simulink model "test_1"  (Simulink 8.9)
settings: Solver=FixedStepAuto  StartTime=0.0  StopTime=inf  RelTol=1e-3  EnableMultiTasking=on
libraries: Solver_SF x1, sldrtlib x1, simulink x1
settings Model: Creator=anan  ModifiedByFormat=an  LastModifiedBy=an
settings DataIOCC: ExternalInput=[t, input_1]  SignalLoggingSaveFormat=Dataset
settings OptimizationCC: ExpressionDepthLimit=2147483647
settings DebuggingCC: SolverPrmCheckMsg=warning

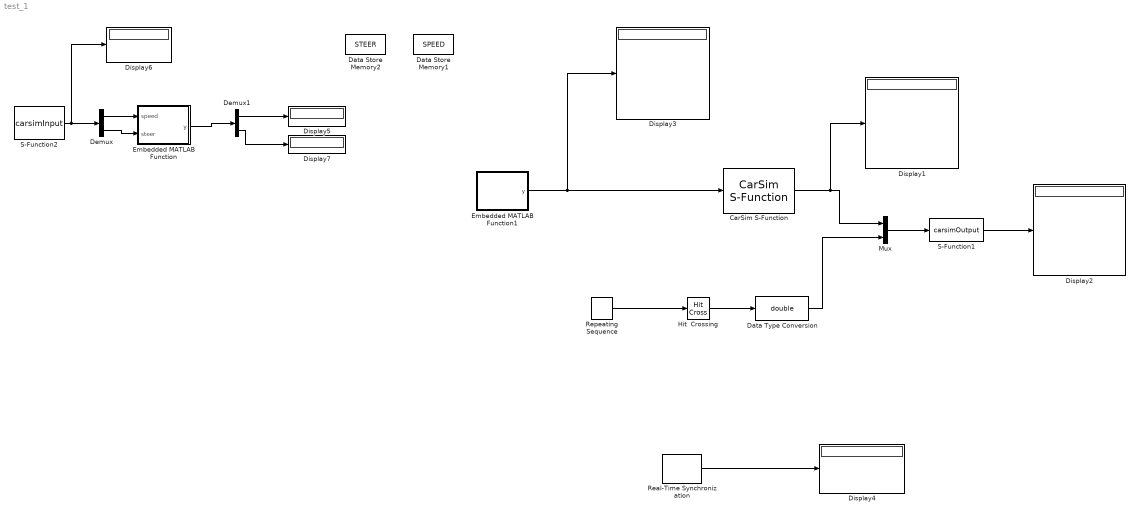
== system test_1 ==
  CarSim S-Function : Solver_SF/CarSim S-Function  Priority=1  VehicleCode=i_s  SIMFILE=simfile.sim
  Data Store Memory1 : DataStoreMemory  DataStoreName=SPEED  ReadBeforeWriteMsg=warning  WriteAfterWriteMsg=warning  WriteAfterReadMsg=warning  ShowAdditionalParam=off  OutDataTypeStr=double
  Data Store Memory2 : DataStoreMemory  DataStoreName=STEER  ReadBeforeWriteMsg=warning  WriteAfterWriteMsg=warning  WriteAfterReadMsg=warning  ShowAdditionalParam=off  OutDataTypeStr=double
  Data Type Conversion : DataTypeConversion  OutDataTypeStr=double
  Demux : Demux  Outputs=2
  Demux1 : Demux  Outputs=2
  Display{1..7} (7 alike) : Display
      Display1 settings: Decimation=2
      Display2 settings: Decimation=2
      Display3 settings: Decimation=2
      Display4 settings: Decimation=2
      Display6 settings: Decimation=2
  Embedded MATLAB Function : MATLAB Function  TreatAsAtomicUnit=on
  Embedded MATLAB Function1 : MATLAB Function  TreatAsAtomicUnit=on
  Hit  Crossing : HitCross  HitCrossingOffset=0.5  HitCrossingDirection=rising
  Mux : Mux  Inputs=2
  Real-Time Synchronization : sldrtlib/Real-Time Synchronization  SampleTime=0.5  MaxMissedTicks=100000  ShowMissedTicks=on  YieldWhenWaiting=on
  Repeating Sequence : simulink/Sources/Repeating Sequence  rep_seq_t=[0 0.01]  rep_seq_y=[0 2]
  S-Function1 : S-Function  FunctionName=carsimOutput  SFunctionDeploymentMode=off  EnableBusSupport=off
  S-Function2 : S-Function  FunctionName=carsimInput  SFunctionDeploymentMode=off  EnableBusSupport=off
  wires:
  S-Function1/1 -> Display2/1
  CarSim S-Function/1 -> Display1/1, Mux/1
  Data Type Conversion/1 -> Mux/2
  Hit  Crossing/1 -> Data Type Conversion/1
  Repeating Sequence/1 -> Hit  Crossing/1
  Real-Time Synchronization/1 -> Display4/1
  Mux/1 -> S-Function1/1
  S-Function2/1 -> Demux/1, Display6/1
  Demux1/2 -> Display7/1
  Embedded MATLAB Function/1(y) -> Demux1/1
  Demux/2 -> Embedded MATLAB Function/2(steer)
  Demux1/1 -> Display5/1
  Demux/1 -> Embedded MATLAB Function/1(speed)
  Embedded MATLAB Function1/1(y) -> Display3/1, CarSim S-Function/1

== matlab function Embedded MATLAB Function1 ==
  data: y output double; SPEED data_store_memory double; STEER data_store_memory double
function y = fcn()
%#eml
global SPEED ;
global STEER ;

y = [SPEED,STEER];

== matlab function Embedded MATLAB Function ==
  data: speed input double; y output double; steer input double; SPEED data_store_memory double; STEER data_store_memory double
function y = fcn(speed,steer)
%#eml
global SPEED ;
global STEER ;
SPEED = speed ;
STEER = steer ;
y = [SPEED,STEER];
